simulink model "BMS_Out"  (R2024a)
settings: Solver=FixedStepDiscrete  StartTime=0.0  StopTime=10000  RelTol=1e-3
model workspace (MAT data in the model file):
  Active_Scenario_Index = Simulink.Parameter
  Active_Scenario_Index.Value = 1
  Active_Scenario_Index.Complexity = 'real'
  Active_Scenario_Index.Dimensions = [1 1]
  Active_Scenario_Index.DataType = 'double'
  BattTempInit = Simulink.Parameter
  BattTempInit.Value = 25
  BattTempInit.Complexity = 'real'
  BattTempInit.Dimensions = [1 1]
  BattTempInit.DataType = 'double'
  Battery.SOC_LUT = [0.01 0.02 0.03 0.04 0.05 0.06 0.07 0.08 0.09 0.1 0.11 0.12 0.13 0.14 0.15 0.16 0.17 0.18 0.19 0.2 0.21 0.22 0.23 0.24 0.25 0.26 0.27 0.28 0.29 0.3 0.31 0.32 0.33 0.34 0.35 0.36 0.37 0.38 0.39 0.4 0.41 0.42 0.43 0.44 0.45 0.46 0.47 0.48 0.49 0.5 0.51 0.52 0.53 0.54 0.55 0.56 0.57 0.58 0.59 0.6 0.61 0.62 0.63 0.64 0.65 0.66 0.67 0.68 0.69 0.7 0.71 0.72 0.73 0.74 0.75 0.76 0.77 0.78 0.79 0.8 0.81 0.82 0.83 0.84 0.85 0.86 0.87 0.88 0.89 0.9 0.91 0.92 0.93 0.94 0.95 0.96 0.97 0.98 0.99 1]
  Battery.Temperature_LUT = [-10 0 25 40]
  Battery.Capacity_LUT = [4.04528301887 4.19622641509 4.8 4.73962264151]
  Battery.Em_LUT = [2.67308083891 2.74411674384 2.80408613071 2.86247711994 2.90851059763 2.94904306488 2.9829846776 3.01467102589 3.04031502638 3.06256828113 3.08180972392 3.09994219643 ... (400 elements, 100x4)]
  Battery.R0_LUT = [0.0569026752707 0.0575506938969 0.0576730924021 0.0575627404981 0.0573787336615 0.0571931123197 0.0568199985482 0.056411926464 0.0561974340667 0.0560805640861 0.0557640899305 0.055275807865 ... (400 elements, 100x4)]
  Battery.R1_LUT = [0.0035 0.0035 0.0035 0.0035 0.0035 0.0035 0.0035 0.0035 0.0035 0.0035 0.0035 0.0035 ... (400 elements, 100x4)]
  Battery.C1_LUT = [5000 5000 5000 5000 5000 5000 5000 5000 5000 5000 5000 5000 ... (400 elements, 100x4)]
  Battery.Mass = 0.047
  Battery.ThermalMass = 44
  Battery.R_bleed = 20
  Battery.h_conv = 5
  Battery.cell_area = 0.0037
  Battery.TempInit = 25
  Battery.SOCInit = 0.75
  Battery.Model = 'panasonic ncr18650bd'
  Battery.DischargeCycle_LUT = [1 5 9 13 17 21 25 29 33 37 41 45 49 53 57 61 65 69 73 77 81 85 89 93 97 101 105 109 113 117 121 125 129 133 137 141 145 149 153 157 161 165 169 173 177 181 185 189 193 197 201 205 209 213 217 221 225 229 233 237 241 245 249 253 257 261 265 269 273 277 281 285 289 293 297 301 305 309 313 317]
  Battery.deltaEm_LUT = [0 -0.363115641304 -0.600096647258 -0.689070000839 -0.76773380251 -0.846397604181 -0.926368385458 -0.992711297521 -1.05704974111 -1.12227693902 -1.19018070587 -1.25808447272 -1.31699459748 -1.35876443799 -1.40168267642 -1.44460091485 -1.48751915327 -1.5304373917 -1.57335563013 -1.62198241593 -1.67232184498 -1.71858340023 -1.76179802551 -1.8050126508 -1.84822727608 -1.8917937136 -1.93575272784 -1.97971174208 -2.02367075632 -2.06762977056 -2.11171979109 -2.15588700406 -2.19980020032 -2.24365853098 -2.28751686164 -2.33137519231 -2.37523352297 -2.41909185363 -2.45982559031 -2.49599372373 -2.53216185715 -2.56832999058 -2.604498124 -2.64066625743 -2.67683439085 -2.71300252428 -2.7491706577 -2.78367585394 -2.81632179346 -2.8483348579 -2.88034792233 -2.91236098677 -2.94437405121 -2.97638711564 -3.00840018008 -3.04041324451 -3.07260346059 -3.10359008254 -3.13082308991 -3.15805609728 -3.18528910464 -3.21252211201 -3.23975511938 -3.26698812675 -3.29422113412 -3.32122400938 -3.3463475604 -3.37152613073 -3.39670470105 -3.42188327138 -3.4470618417 -3.47224041203 -3.49938358795 -3.52900276724 -3.55862194653 -3.58824112582 -3.6178603051 -3.64748858268 -3.67711690909 -3.70674523549]
  Battery.deltaCapacity_LUT = [0 -0.860019120059 -1.71332421702 -2.0819400264 -2.45055583577 -2.81917164515 -3.18778745452 -3.48884924257 -3.7808148236 -4.07278040463 -4.36474598566 -4.6567115667 -4.91000721732 -5.08494410056 -5.2598809838 -5.43481786703 -5.60975475027 -5.78469163351 -5.95962851674 -6.13456539998 -6.30950228322 -6.47026795816 -6.62044510558 -6.77062225299 -6.92079940041 -7.07097654783 -7.22115369524 -7.37133084266 -7.52150799007 -7.67168513749 -7.82230984162 -7.97319825819 -8.12408667477 -8.27497509134 -8.42586350792 -8.57675192449 -8.72764034107 -8.87852875764 -9.01789522921 -9.13717923376 -9.25646323831 -9.37574724285 -9.4950312474 -9.61431525195 -9.73359925649 -9.85288326104 -9.97216726558 -10.0914512701 -10.2059878191 -10.3183039593 -10.4306200996 -10.5429362398 -10.65525238 -10.7675685203 -10.8798846605 -10.9922008008 -11.104516941 -11.2125891929 -11.3075699376 -11.4025506823 -11.4975314271 -11.5925121718 -11.6874929166 -11.7824736613 -11.877454406 -11.9716325175 -12.0588579537 -12.1460833899 -12.2333088261 -12.3205342623 -12.4077596986 -12.4949851348 -12.5890165008 -12.6916254178 -12.7942343349 -12.8968432519 -12.999452169 -13.102061086 -13.2046700031 -13.3072789201]
  Battery.cond_thickness = 0.001
  Battery.thermal_conductivity = 205
  CellType = Simulink.Parameter
  CellType.Value = 1
  CellType.Complexity = 'real'
  CellType.Dimensions = [1 1]
  CellType.DataType = 'double'
  Np_Module = Simulink.Parameter
  Np_Module.Value = 31
  Np_Module.Complexity = 'real'
  Np_Module.Dimensions = [1 1]
  Np_Module.DataType = 'double'
  Ns_Module = Simulink.Parameter
  Ns_Module.Value = 24
  Ns_Module.Complexity = 'real'
  Ns_Module.Dimensions = [1 1]
  Ns_Module.DataType = 'double'
  NumModules = Simulink.Parameter
  NumModules.Value = 4
  NumModules.Complexity = 'real'
  NumModules.Dimensions = [1 1]
  NumModules.DataType = 'double'
  OverCellVoltageLimit = Simulink.Parameter
  OverCellVoltageLimit.Value = 4.19999980927
  OverCellVoltageLimit.Complexity = 'real'
  OverCellVoltageLimit.Dimensions = [1 1]
  OverCellVoltageLimit.DataType = 'single'
  TestCase = Simulink.Parameter
  TestCase.Value = 1
  TestCase.Complexity = 'real'
  TestCase.Dimensions = [1 1]
  TestCase.DataType = 'double'
  UnderCellVoltageLimit = Simulink.Parameter
  UnderCellVoltageLimit.Value = 2.5
  UnderCellVoltageLimit.Complexity = 'real'
  UnderCellVoltageLimit.Dimensions = [1 1]
  UnderCellVoltageLimit.DataType = 'single'
  ts = Simulink.Parameter
  ts.Value = 0.1
  ts.Complexity = 'real'
  ts.Dimensions = [1 1]
  ts.DataType = 'double'
settings Model: DataDictionary=DD_BMS_Out.sldd  ModifiedByFormat=The MathWorks, Inc.  ExtModeTrigDuration=5  Creator=The MathWorks, Inc.  LastModifiedBy=The MathWorks, Inc.
settings SolverCC: AlgebraicLoopSolver=TrustRegion  PositivePriorityOrder=on  AutoInsertRateTranBlk=on  MaxZcPerStep=1
settings DataIOCC: ExternalInput=Battery  SaveOutput=off  SaveTime=off  SignalLoggingName=logsOut
settings OptimizationCC: BlockReduction=off  DefaultParameterBehavior=Inlined  UseFloatMulNetSlope=on  DefaultUnderspecifiedDataType=single  OptimizeBlockIOStorage=off  EnhancedBackFolding=on  PassReuseOutputArgsThreshold=0  EfficientFloat2IntCast=on  MaxStackSize=64  OptimizeBlockOrder=speed  DifferentSizesBufferReuse=on
settings DebuggingCC: SignalInfNanChecking=error  SaveWithParameterizedLinksMsg=none  CheckExecutionContextPreStartOutputMsg=on  IntegerOverflowMsg=error  ParameterPrecisionLossMsg=none  ParameterTunabilityLossMsg=error  UnconnectedInputMsg=warning  UnconnectedOutputMsg=warning  UnconnectedLineMsg=warning  AssertControl=DisableAll  AllowSymbolicDim=off  PregeneratedLibrarySubsystemCodeDiagnostic=none  SFUnexpectedBacktrackingDiag=warning  SFNoUnconditionalDefaultTransitionDiag=warning  SFExecutionAtInitializationDiag=none  ArithmeticOperatorsInVariantConditions=warning
settings ModelReferenceCC: EnableRefExpFcnMdlSchedulingChecks=on  ModelReferenceNumInstancesAllowed=Single  PropagateSignalLabelsOutOfModel=off
settings SFSimCC: SimUseLocalCustomCode=off  MATLABDynamicMemAlloc=off  CustomCodeUndefinedFunction=UseInterfaceOnly
settings RTWCC: GenerateReport=on  RTWUseLocalCustomCode=off  GPUComputeCapability=3.5  DLArmComputeVersion=19.05
settings CodeAppCC: ForceParamTrailComments=on  MaxIdLength=51  OperatorAnnotations=on  MangleLength=4
settings GRTTargetCC: TargetLangStandard=C89/C90 (ANSI)
settings ConfigComp: CovMetricSettings=dcw  CovSaveCumulativeToWorkspaceVar=on  CovSaveSingleToWorkspaceVar=on  CovExternalEMLEnable=off  CovSFcnEnable=off  DVMode=DesignErrorDetection  DVMaxProcessTime=7000  DVTestSuiteOptimization=Auto  DVDetectDeadLogic=on  DVDetectIntegerOverflow=off  DVRebuildModelRepresentation=Always

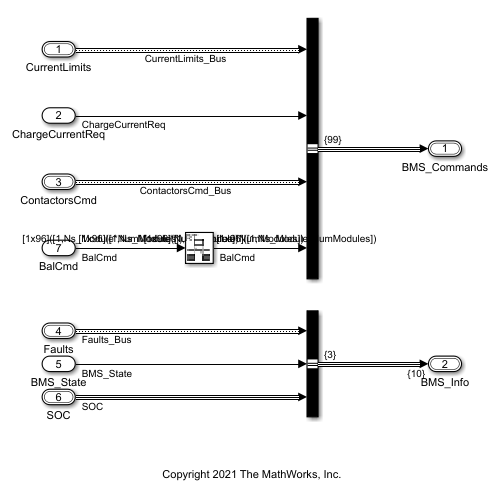
[thumbnail: Simulink's stored preview of the top-level diagram]
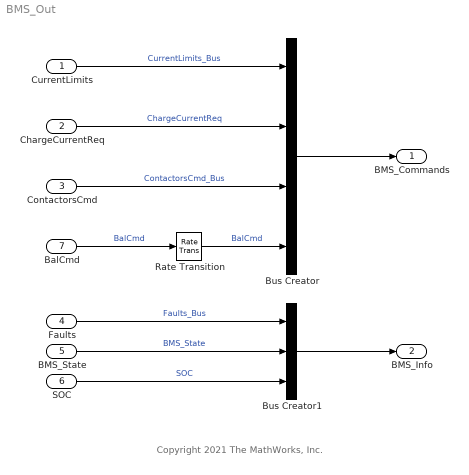
== system BMS_Out ==
  note: Copyright 2021 The MathWorks, Inc.
  CurrentLimits : Inport  OutDataTypeStr=Bus: CurrentLimits  SampleTime=[0.10000000000000001,0]  BusOutputAsStruct=on
  ChargeCurrentReq : Inport  Port=2  OutDataTypeStr=single  PortDimensions=1  SampleTime=[0.10000000000000001,0]
  ContactorsCmd : Inport  Port=3  OutDataTypeStr=Bus: Contactors_Cmd  SampleTime=[0.10000000000000001,0]  BusOutputAsStruct=on
  Faults : Inport  Port=4  OutDataTypeStr=Bus: Faults  PortDimensions=1  SampleTime=[0.10000000000000001,0]  BusOutputAsStruct=on
  BMS_State : Inport  Port=5  OutDataTypeStr=Enum: BMS_State_Enum  PortDimensions=1  SampleTime=[0.10000000000000001,0]
  SOC : Inport  Port=6  OutDataTypeStr=Bus: SOC_Est  SampleTime=[0.10000000000000001,0]
  BalCmd : Inport  Port=7  OutDataTypeStr=boolean  PortDimensions=[1 NumModules*Ns_Module]  SampleTime=[5,0]
  Bus Creator1 : BusCreator  Inputs=3  OutDataTypeStr=Bus: BMS_Info
  Bus Creator : BusCreator  Inputs=4  OutDataTypeStr=Bus: BMS_Cmd
  Rate Transition : RateTransition  Integrity=off  Deterministic=off
  BMS_Commands : Outport  OutDataTypeStr=Bus: BMS_Cmd  SampleTime=[0.10000000000000001,0]  BusOutputAsStruct=on
  BMS_Info : Outport  Port=2  OutDataTypeStr=Bus: BMS_Info  SampleTime=[0.10000000000000001,0]
  wires:
  ContactorsCmd/1 -> Bus Creator/3  "ContactorsCmd_Bus"
  Faults/1 -> Bus Creator1/1  "Faults_Bus"
  Bus Creator1/1 -> BMS_Info/1
  BalCmd/1 -> Rate Transition/1  "BalCmd"
  Bus Creator/1 -> BMS_Commands/1
  SOC/1 -> Bus Creator1/3  "SOC"
  BMS_State/1 -> Bus Creator1/2  "BMS_State"
  CurrentLimits/1 -> Bus Creator/1  "CurrentLimits_Bus"
  ChargeCurrentReq/1 -> Bus Creator/2  "ChargeCurrentReq"
  Rate Transition/1 -> Bus Creator/4  "BalCmd"
